simulink model "counter_test_16_ip"  (Simulink 6.2)
settings: Solver=ode45  StartTime=0.0  StopTime=6000  RelTol=1e-3
undefined symbols (not defined in the file or in its folder): iBOB
libraries: xbsIndex_r3 x81, xps_library x42, casper_library x11
settings Model: LastModifiedBy=tfiliba
settings DebuggingCC: SolverPrmCheckMsg=warning

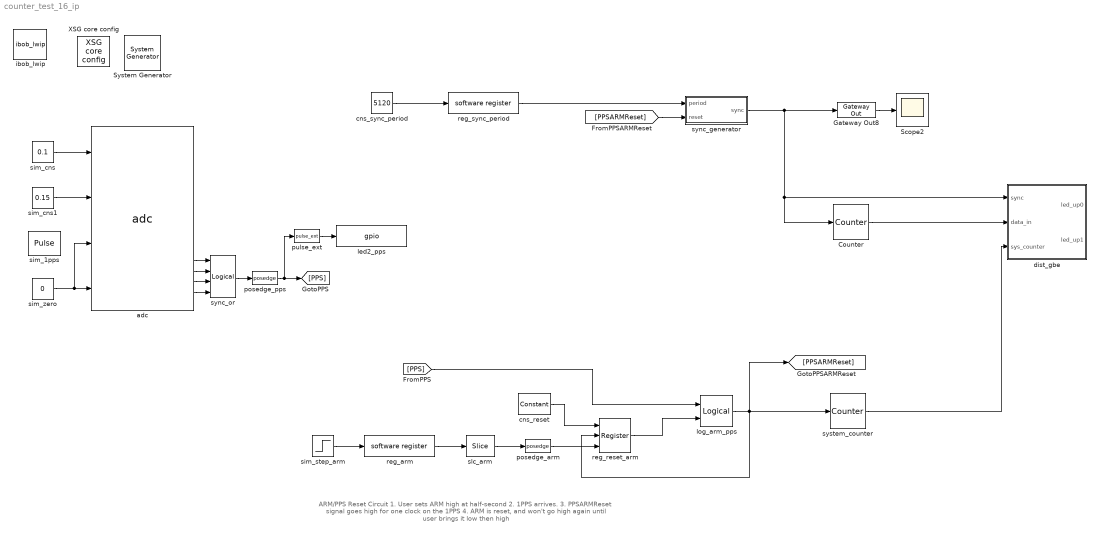
== system counter_test_16_ip ==
  note: ARM/PPS Reset Circuit
      | 1. User sets ARM high at half-second
      | 2. 1PPS arrives.
      | 3. PPSARMReset signal goes high for one clock on the 1PPS
      | 4. ARM is reset, and won't go high again until user brings it low then high
  " System Generator" : xbsIndex_r3/ System Generator  Tag=genX  xilinxfamily=Virtex2P  part=xc2vp50  speed=-7  package=ff1152  synthesis_tool=XST  directory=./counter_test_16_ip/sysgen  testbench=off  simulink_period=1  sysclk_period=5  incr_netlist=off  trim_vbits=Everywhere in SubSystem  dbl_ovrd=According to Block Masks  core_generation=According to Block Masks  run_coregen=off  deprecated_control=off  eval_field=0
      settings: AttributesFormatString=System\nGenerator
  Counter : xbsIndex_r3/Counter  cnt_type=Count Limited  n_bits=64  bin_pt=0  arith_type=Unsigned  start_count=0  cnt_to=15  cnt_by_val=1  operation=Up  explicit_period=on  period=1  load_pin=off  rst=on  en=off  dbl_ovrd=off  show_param=off  use_rpm=on  gen_core=off
      settings: xl_area=[0, 0, 0, 0, 0, 0, 0]
  Gateway Out8 : xbsIndex_r3/Gateway Out  output_type=Double  nbits=8  bin_pt=6  arith_type=Boolean  quantization=Truncate  overflow=Wrap  hdl_port=on  timing_constraint=None  locs_specified=off  LOCs={}  needs_fixed_name=off  show_param=off
      settings: xl_area=[0, 0, 0, 0, 0, 0, 0]
  Scope2 : Scope
      settings: YMin=-1  YMax=1  SaveName=ScopeData3
  XSG core config : xps_library/XSG core config  Tag=xps:xsg  hw_sys=iBOB  ibob_linux=off  clk_src=adc0_clk  gpio_clk_io_group=iBOB:sma  gpio_clk_bit_index=0  clk_rate=200  sample_period=1  synthesis_tool=XST  mpc_type=powerpc405
  adc : xps_library/adc  Tag=xps:adc  adc_brd=iBOB:adc0  adc_clk_rate=800  adc_interleave=off  sample_period=1
  cns_reset : xbsIndex_r3/Constant  const=1  equ=P=C  arith_type=Boolean  n_bits=1  bin_pt=0  opselect=C  inp2=PCIN>>17  opr=+  inp1=P  carry=CIN  iostate=0  explicit_period=on  period=1  dbl_ovrd=off
  cns_sync_period : Constant  Value=5120
  dist_gbe : Subsystem  mask(dist_gbe){numcomputers=16, numsamples=16, samplesperpacket=64}
      mask prompts: numcomputers "Num IPs (Must be power of 2)"; numsamples "Samples per spectrum (Number of clock cycles to generate 1 spectrum)"; samplesperpacket "Samples per packet (Number of samples to put in a packet)"
      mask init:
      | dist_gbe_init(gcb,...
      |     'numcomputers', numcomputers,...
      |     'numsamples', numsamples,...
      |     'samplesperpacket', samplesperpacket)
      settings: AttributesFormatString=IPs=16
  ibob_lwip : xps_library/ibob_lwip
  led2_pps : xps_library/gpio  Tag=xps:gpio  io_group=iBOB:led  io_dir=out  arith_type=Boolean  bitwidth=1  bin_pt=0  bit_index=3  sample_period=1  use_single_ended=off  use_ddr=off  reg_iob=on  reg_clk_phase=0  termination=None
  log_arm_pps : xbsIndex_r3/Logical  logical_function=AND  inputs=2  precision=Full  arith_type=Unsigned  n_bits=8  bin_pt=2  align_bp=on  latency=0  explicit_period=off  period=1  en=off  dbl_ovrd=off  show_param=off
      settings: xl_area=[0, 0, 0, 0, 0, 0, 0]
  posedge_arm : casper_library/Misc/posedge  Tag=Rising Edge Detector
  posedge_pps : casper_library/Misc/posedge  Tag=Rising Edge Detector
  pulse_ext : casper_library/Misc/pulse_ext  pulse_len=10000000
  reg_arm : xps_library/software register  Tag=xps:sw_reg  io_dir=From Processor  arith_type=Unsigned  bitwidth=32  bin_pt=0  sample_period=1  gw_name=counter_test_16_ip_reg_arm_user_data_out
  reg_reset_arm : xbsIndex_r3/Register  init=0  reg_only_valid=off  explicit_period=on  period=1  rst=on  en=on  out_en=off  dbl_ovrd=off  show_param=off
      settings: xl_area=[0, 0, 0, 0, 0, 0, 0]
  reg_sync_period : xps_library/software register  Tag=xps:sw_reg  io_dir=From Processor  arith_type=Unsigned  bitwidth=32  bin_pt=0  sample_period=1  gw_name=counter_test_16_ip_reg_sync_period_user_data_out
  sim_1pps : DiscretePulseGenerator  Period=1000  PulseWidth=3
  sim_cns : Constant  Value=0.1
  sim_cns1 : Constant  Value=0.15
  sim_step_arm : Step  SampleTime=0
  sim_zero : Constant  Value=0
  slc_arm : xbsIndex_r3/Slice  mode=Lower Bit Location + Width  nbits=1  bit1=0  base1=MSB of Input  bit0=0  base0=LSB of Input  boolean_output=on  explicit_period=off  period=1  dbl_ovrd=off
  sync_generator : Subsystem
  sync_or : xbsIndex_r3/Logical  logical_function=OR  inputs=4  precision=Full  arith_type=Unsigned  n_bits=8  bin_pt=2  align_bp=on  latency=1  explicit_period=off  period=1  en=off  dbl_ovrd=off  show_param=off
      settings: xl_area=[0, 0, 0, 0, 0, 0, 0]
  system_counter : xbsIndex_r3/Counter  cnt_type=Free Running  n_bits=64  bin_pt=0  arith_type=Unsigned  start_count=0  cnt_to=Inf  cnt_by_val=1  operation=Up  explicit_period=off  period=1  load_pin=off  rst=on  en=off  dbl_ovrd=off  show_param=off  use_rpm=on  gen_core=off
      settings: xl_area=[0, 0, 0, 0, 0, 0, 0]
  wires:
  reg_arm/1 -> slc_arm/1
  cns_reset/1 -> reg_reset_arm/1
  reg_reset_arm/1 -> log_arm_pps/2
  [PPS] -> log_arm_pps/1
  log_arm_pps/1 -> reg_reset_arm/2, system_counter/1, [PPSARMReset]
  slc_arm/1 -> posedge_arm/1
  posedge_arm/1 -> reg_reset_arm/3
  sim_step_arm/1 -> reg_arm/1
  reg_sync_period/1 -> sync_generator/1(period)
  sync_generator/1(sync) -> Gateway Out8/1, Counter/1, dist_gbe/1(sync)
  cns_sync_period/1 -> reg_sync_period/1
  Gateway Out8/1 -> Scope2/1
  [PPSARMReset] -> sync_generator/2(reset)
  sim_zero/1 -> adc/4, adc/3
  adc/13 -> sync_or/1
  adc/14 -> sync_or/2
  adc/15 -> sync_or/3
  adc/16 -> sync_or/4
  sync_or/1 -> posedge_pps/1
  posedge_pps/1 -> [PPS], pulse_ext/1
  pulse_ext/1 -> led2_pps/1
  sim_cns/1 -> adc/1
  sim_cns1/1 -> adc/2
  Counter/1 -> dist_gbe/2(data_in)
  system_counter/1 -> dist_gbe/3(sys_counter)

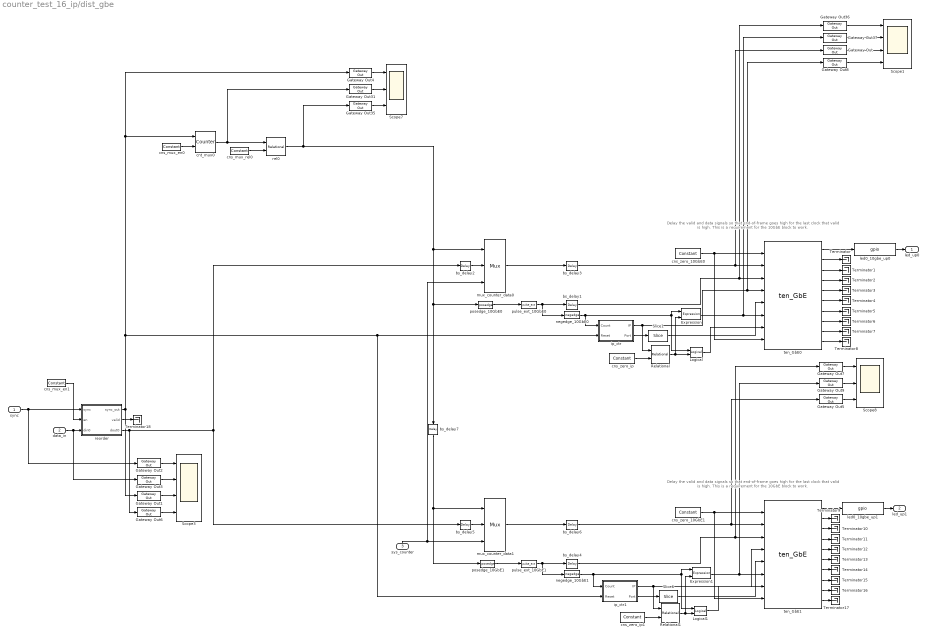
== system counter_test_16_ip/dist_gbe ==
  note: Delay the valid and data signals so that
      | end-of-frame goes high for the last clock
      | that valid is high. This is a requirement for
      | the 10GbE block to work.
  note: Delay the valid and data signals so that
      | end-of-frame goes high for the last clock
      | that valid is high. This is a requirement for
      | the 10GbE block to work.
  sync : Inport  Port=1  LatchInput=off
  data_in : Inport  Port=2  LatchInput=off
  sys_counter : Inport  Orientation=up  Port=3  LatchInput=off
  Expression : xbsIndex_r3/Expression  expression=a & ~b  precision=Full  arith_type=Unsigned  n_bits=8  bin_pt=2  align_bp=on  latency=0  explicit_period=off  period=1  en=off  dbl_ovrd=off  show_param=off
      settings: xl_area=[0, 0, 0, 0, 0, 0, 0]
  Expression1 : xbsIndex_r3/Expression  expression=a & ~b  precision=Full  arith_type=Unsigned  n_bits=8  bin_pt=2  align_bp=on  latency=0  explicit_period=off  period=1  en=off  dbl_ovrd=off  show_param=off
      settings: xl_area=[0, 0, 0, 0, 0, 0, 0]
  Gateway Out{,1..9,31,35..37} (14 alike) : xbsIndex_r3/Gateway Out  output_type=Double  nbits=8  bin_pt=6  arith_type=Boolean  quantization=Truncate  overflow=Wrap  hdl_port=on  timing_constraint=None  locs_specified=off  LOCs={}  needs_fixed_name=off  show_param=off
      settings: xl_area=[0, 0, 0, 0, 0, 0, 0]
  Logical : xbsIndex_r3/Logical  logical_function=AND  inputs=2  precision=Full  arith_type=Unsigned  n_bits=8  bin_pt=2  align_bp=on  latency=0  explicit_period=off  period=1  en=off  dbl_ovrd=off  show_param=off
      settings: xl_area=[0, 0, 0, 0, 0, 0, 0]
  Logical1 : xbsIndex_r3/Logical  logical_function=AND  inputs=2  precision=Full  arith_type=Unsigned  n_bits=8  bin_pt=2  align_bp=on  latency=0  explicit_period=off  period=1  en=off  dbl_ovrd=off  show_param=off
      settings: xl_area=[0, 0, 0, 0, 0, 0, 0]
  Relational : xbsIndex_r3/Relational  mode=a=b  latency=0  explicit_period=off  period=1  en=off  dbl_ovrd=off  show_param=off
      settings: xl_area=[0, 0, 0, 0, 0, 0, 0]
  Relational1 : xbsIndex_r3/Relational  mode=a=b  latency=0  explicit_period=off  period=1  en=off  dbl_ovrd=off  show_param=off
      settings: xl_area=[0, 0, 0, 0, 0, 0, 0]
  Scope1 : Scope  NumInputPorts=4
      settings: TimeRange=10000  YMin=0~0~-5~-5  YMax=1~1~40~5
  Scope3 : Scope  NumInputPorts=4
      settings: TimeRange=6000  YMin=0~0~-1~0  YMax=1~65~1~65  SaveName=ScopeData4
  Scope7 : Scope  NumInputPorts=3
      settings: YMin=0~0~0  YMax=1~275~1
  Scope8 : Scope  NumInputPorts=3
      settings: TimeRange=6000  YMin=0~0~0  YMax=1~1~5250  SaveName=ScopeData2
  Slice1 : xbsIndex_r3/Slice  mode=Lower Bit Location + Width  nbits=16  bit1=0  base1=MSB of Input  bit0=0  base0=LSB of Input  boolean_output=off  explicit_period=off  period=1  dbl_ovrd=off
  Slice6 : xbsIndex_r3/Slice  mode=Lower Bit Location + Width  nbits=16  bit1=0  base1=MSB of Input  bit0=0  base0=LSB of Input  boolean_output=off  explicit_period=off  period=1  dbl_ovrd=off
  Terminator{,1..18} (19 alike) : Terminator
  bs_delay{1..6} (6 alike) : xbsIndex_r3/Delay  latency=1  reg_retiming=off  explicit_period=on  period=1  en=off  accept_only_valid=off  init_zero=on  dbl_ovrd=off  show_param=off
      settings: xl_area=[0, 0, 0, 0, 0, 0, 0]
  bs_delay7 : xbsIndex_r3/Delay  Orientation=down  latency=64  reg_retiming=off  explicit_period=on  period=1  en=off  accept_only_valid=off  init_zero=on  dbl_ovrd=off  show_param=off
      settings: xl_area=[0, 0, 0, 0, 0, 0, 0]
  cns_mux_en0 : xbsIndex_r3/Constant  const=1  equ=P=C  arith_type=Boolean  n_bits=1  bin_pt=0  opselect=C  inp2=PCIN>>17  opr=+  inp1=P  carry=CIN  iostate=0  explicit_period=on  period=1  dbl_ovrd=off
  cns_mux_en1 : xbsIndex_r3/Constant  const=1  equ=P=C  arith_type=Boolean  n_bits=1  bin_pt=0  opselect=C  inp2=PCIN>>17  opr=+  inp1=P  carry=CIN  iostate=0  explicit_period=on  period=1  dbl_ovrd=off
  cns_mux_rel0 : xbsIndex_r3/Constant  const=127  equ=P=C  arith_type=Unsigned  n_bits=7  bin_pt=0  opselect=C  inp2=PCIN>>17  opr=+  inp1=P  carry=CIN  iostate=0  explicit_period=on  period=1  dbl_ovrd=off
  cns_zero_10GbE0 : xbsIndex_r3/Constant  const=0  equ=P=C  arith_type=Boolean  n_bits=32  bin_pt=0  opselect=C  inp2=PCIN>>17  opr=+  inp1=P  carry=CIN  iostate=0  explicit_period=on  period=1  dbl_ovrd=off
  cns_zero_10GbE1 : xbsIndex_r3/Constant  const=0  equ=P=C  arith_type=Boolean  n_bits=32  bin_pt=0  opselect=C  inp2=PCIN>>17  opr=+  inp1=P  carry=CIN  iostate=0  explicit_period=on  period=1  dbl_ovrd=off
  cns_zero_ip : xbsIndex_r3/Constant  const=0  equ=P=C  arith_type=Unsigned  n_bits=32  bin_pt=0  opselect=C  inp2=PCIN>>17  opr=+  inp1=P  carry=CIN  iostate=0  explicit_period=on  period=1  dbl_ovrd=off
  cns_zero_ip1 : xbsIndex_r3/Constant  const=0  equ=P=C  arith_type=Unsigned  n_bits=32  bin_pt=0  opselect=C  inp2=PCIN>>17  opr=+  inp1=P  carry=CIN  iostate=0  explicit_period=on  period=1  dbl_ovrd=off
  cnt_mux0 : xbsIndex_r3/Counter  cnt_type=Free Running  n_bits=7  bin_pt=0  arith_type=Unsigned  start_count=0  cnt_to=Inf  cnt_by_val=1  operation=Up  explicit_period=off  period=1  load_pin=off  rst=on  en=on  dbl_ovrd=off  show_param=off  use_rpm=on  gen_core=off
      settings: xl_area=[0, 0, 0, 0, 0, 0, 0]
  ip_ctr : Subsystem  mask(ip_ctr){numcomputers=8, odd_channels=1}
      mask prompts: numcomputers "Num IPs (Must be power of 2)"; odd_channels "Odd Channels"
      mask init:
      | ip_ctr_init(gcb,...
      |     'numcomputers',numcomputers,...
      |     'odd_channels',odd_channels)
      settings: AttributesFormatString=IPs=8
  ip_ctr1 : Subsystem  mask(ip_ctr){numcomputers=8, odd_channels=0}
      mask prompts: numcomputers "Num IPs (Must be power of 2)"; odd_channels "Odd Channels"
      mask init:
      | ip_ctr_init(gcb,...
      |     'numcomputers',numcomputers,...
      |     'odd_channels',odd_channels)
      settings: AttributesFormatString=IPs=8
  led0_10gbe_up0 : xps_library/gpio  Tag=xps:gpio  io_group=iBOB:led  io_dir=out  arith_type=Boolean  bitwidth=1  bin_pt=0  bit_index=1  sample_period=1  use_single_ended=off  use_ddr=off  reg_iob=on  reg_clk_phase=0  termination=None
  led0_10gbe_up1 : xps_library/gpio  Tag=xps:gpio  io_group=iBOB:led  io_dir=out  arith_type=Boolean  bitwidth=1  bin_pt=0  bit_index=2  sample_period=1  use_single_ended=off  use_ddr=off  reg_iob=on  reg_clk_phase=0  termination=None
  mux_counter_data0 : xbsIndex_r3/Mux  inputs=2  precision=Full  arith_type="Signed  (2's comp)"  n_bits=8  bin_pt=2  quantization=Truncate  overflow=Wrap  latency=1  explicit_period=off  period=1  en=off  dbl_ovrd=off  show_param=off  mux_type=off  use_rpm=off  gen_core=off
      settings: xl_area=[0, 0, 0, 0, 0, 0, 0]
  mux_counter_data1 : xbsIndex_r3/Mux  inputs=2  precision=Full  arith_type="Signed  (2's comp)"  n_bits=8  bin_pt=2  quantization=Truncate  overflow=Wrap  latency=1  explicit_period=off  period=1  en=off  dbl_ovrd=off  show_param=off  mux_type=off  use_rpm=off  gen_core=off
      settings: xl_area=[0, 0, 0, 0, 0, 0, 0]
  negedge_10GbE0 : casper_library/Misc/negedge  Tag=Rising Edge Detector
  negedge_10GbE1 : casper_library/Misc/negedge  Tag=Rising Edge Detector
  posedge_10GbE0 : casper_library/Misc/posedge  Tag=Rising Edge Detector
  posedge_10GbE1 : casper_library/Misc/posedge  Tag=Rising Edge Detector
  pulse_ext_10GbE0 : casper_library/Misc/pulse_ext  pulse_len=65
  pulse_ext_10GbE1 : casper_library/Misc/pulse_ext  pulse_len=65
  rel0 : xbsIndex_r3/Relational  mode=a=b  latency=1  explicit_period=off  period=1  en=off  dbl_ovrd=off  show_param=off
      settings: xl_area=[0, 0, 0, 0, 0, 0, 0]
  reorder : Subsystem  AncestorBlock=casper_library/Reorder/reorder  mask(reorder){map=[0 16 32 48 64 80 96 112 128 144 160 176 192 208 224 240 256 272 288 304 320 336 352 368 384 400 416 432 448 464 480 496 512 528 544 560 576 592 608 624 640 656 672 688 704 720 736 752 768 784 800 816 832 848 864 880 896 912 928 944 960 976 992 1008 1 17 33 49 65 81 97 113 129 145 161 177 193 209 225 241 257 273 289 305 321 337 353 369 385 401 417 433 449 465 481 497 513 529 545 561 577 593 609 625 641 657 673 689 705 721 737 753 769 785 801 817 833 849 865 881 897 913 929 945 961 977 993 1009 2 18 34 50 66 82 98 114 130 146 162 178 194 210 226 242 258 274 290 306 322 338 354 370 386 402 418 434 450 466 482 498 514 530 546 562 578 594 610 626 642 658 674 690 706 722 738 754 770 786 802 818 834 850 866 882 898 914 930 946 962 978 994 1010 3 19 35 51 67 83 99 115 131 147 163 179 195 211 227 243 259 275 291 307 323 339 355 371 387 403 419 435 451 467 483 499 515 531 547 563 579 595 611 627 643 659 675 691 707 723 739 755 771 787 803 819 835 851 867 883 899 915 931 947 963 979 995 1011 4 20 36 52 68 84 100 116 132 148 164 180 196 212 228 244 260 276 292 308 324 340 356 372 388 404 420 436 452 468 484 500 516 532 548 564 580 596 612 628 644 660 676 692 708 724 740 756 772 788 804 820 836 852 868 884 900 916 932 948 964 980 996 1012 5 21 37 53 69 85 101 117 133 149 165 181 197 213 229 245 261 277 293 309 325 341 357 373 389 405 421 437 453 469 485 501 517 533 549 565 581 597 613 629 645 661 677 693 709 725 741 757 773 789 805 821 837 853 869 885 901 917 933 949 965 981 997 1013 6 22 38 54 70 86 102 118 134 150 166 182 198 214 230 246 262 278 294 310 326 342 358 374 390 406 422 438 454 470 486 502 518 534 550 566 582 598 614 630 646 662 678 694 710 726 742 758 774 790 806 822 838 854 870 886 902 918 934 950 966 982 998 1014 7 23 39 55 71 87 103 119 135 151 167 183 199 215 231 247 263 279 295 311 327 343 359 375 391 407 423 439 455 471 487 503 519 535 551 567 583 599 615 631 647 663 679 695 711 727 743 759 775 791 807 823 839 855 871 887 903 919 935 951 967 983 999 1015 8 24 40 56 72 88 104 120 136 152 168 184 200 216 232 248 264 280 296 312 328 344 360 376 392 408 424 440 456 472 488 504 520 536 552 568 584 600 616 632 648 664 680 696 712 728 744 760 776 792 808 824 840 856 872 888 904 920 936 952 968 984 1000 1016 9 25 41 57 73 89 105 121 137 153 169 185 201 217 233 249 265 281 297 313 329 345 361 377 393 409 425 441 457 473 489 505 521 537 553 569 585 601 617 633 649 665 681 697 713 729 745 761 777 793 809 825 841 857 873 889 905 921 937 953 969 985 1001 1017 10 26 42 58 74 90 106 122 138 154 170 186 202 218 234 250 266 282 298 314 330 346 362 378 394 410 426 442 458 474 490 506 522 538 554 570 586 602 618 634 650 666 682 698 714 730 746 762 778 794 810 826 842 858 874 890 906 922 938 954 970 986 1002 1018 11 27 43 59 75 91 107 123 139 155 171 187 203 219 235 251 267 283 299 315 331 347 363 379 395 411 427 443 459 475 491 507 523 539 555 571 587 603 619 635 651 667 683 699 715 731 747 763 779 795 811 827 843 859 875 891 907 923 939 955 971 987 1003 1019 12 28 44 60 76 92 108 124 140 156 172 188 204 220 236 252 268 284 300 316 332 348 364 380 396 412 428 444 460 476 492 508 524 540 556 572 588 604 620 636 652 668 684 700 716 732 748 764 780 796 812 828 844 860 876 892 908 924 940 956 972 988 1004 1020 13 29 45 61 77 93 109 125 141 157 173 189 205 221 237 253 269 285 301 317 333 349 365 381 397 413 429 445 461 477 493 509 525 541 557 573 589 605 621 637 653 669 685 701 717 733 749 765 781 797 813 829 845 861 877 893 909 925 941 957 973 989 1005 1021 14 30 46 62 78 94 110 126 142 158 174 190 206 222 238 254 270 286 302 318 334 350 366 382 398 414 430 446 462 478 494 510 526 542 558 574 590 606 622 638 654 670 686 702 718 734 750 766 782 798 814 830 846 862 878 894 910 926 942 958 974 990 1006 1022 15 31 47 63 79 95 111 127 143 159 175 191 207 223 239 255 271 287 303 319 335 351 367 383 399 415 431 447 463 479 495 511 527 543 559 575 591 607 623 639 655 671 687 703 719 735 751 767 783 799 815 831 847 863 879 895 911 927 943 959 975 991 1007 1023], n_inputs=1, bram_latency=2, map_latency=1, double_buffer=0}
      mask prompts: map "Output Order:"; n_inputs "Number of inputs"; bram_latency "BRAM Latency"; map_latency "Map Latency"; double_buffer "Double Buffer"
      mask init:
      | reorder_init(gcb, ...
      |     'map', map, ...
      |     'n_inputs', n_inputs, ...
      |     'bram_latency', bram_latency, ...
      |     'map_latency', map_latency, ...
      |     'double_buffer', double_buffer);
      settings: AttributesFormatString=order=5
  ten_GbE0 : xps_library/ten_GbE  Tag=xps:tengbe  port=iBOB:0  mac_lite=on  show_param=on  pre_emph=2  swing=800
  ten_GbE1 : xps_library/ten_GbE  Tag=xps:tengbe  port=iBOB:1  mac_lite=on  show_param=on  pre_emph=2  swing=800
  led_up0 : Outport
  led_up1 : Outport  Port=2
  wires:
  sys_counter/1 -> mux_counter_data1/3, mux_counter_data0/3
  data_in/1 -> Gateway Out3/1, reorder/3(din0)
  reorder/2(valid) -> Terminator18/1
  Gateway Out36/1 -> Scope1/1
  ten_GbE1/10 -> Terminator17/1
  ten_GbE1/9 -> Terminator16/1
  ten_GbE1/8 -> Terminator15/1
  ten_GbE1/7 -> Terminator14/1
  ten_GbE1/6 -> Terminator13/1
  ten_GbE1/5 -> Terminator12/1
  ten_GbE1/4 -> Terminator11/1
  ten_GbE1/3 -> Terminator10/1
  ten_GbE1/2 -> Terminator9/1
  ten_GbE0/10 -> Terminator8/1
  ten_GbE0/9 -> Terminator7/1
  ten_GbE0/8 -> Terminator6/1
  ten_GbE0/7 -> Terminator5/1
  ten_GbE0/6 -> Terminator4/1
  ten_GbE0/5 -> Terminator3/1
  ten_GbE0/4 -> Terminator2/1
  ten_GbE0/3 -> Terminator1/1
  ten_GbE0/2 -> Terminator/1
  ten_GbE0/1 -> led0_10gbe_up0/1
  cns_zero_10GbE0/1 -> ten_GbE0/1, ten_GbE0/8
  mux_counter_data0/1 -> bs_delay3/1
  cnt_mux0/1 -> rel0/1, Gateway Out31/1
  cns_mux_en0/1 -> cnt_mux0/2
  Gateway Out37/1 -> Scope1/2
  Gateway Out/1 -> Scope1/3
  pulse_ext_10GbE0/1 -> bs_delay1/1, negedge_10GbE0/1
  negedge_10GbE0/1 -> Logical/1, Expression/1, ip_ctr/1(Count)
  cns_mux_rel0/1 -> rel0/2
  rel0/1 -> mux_counter_data0/1, posedge_10GbE0/1, bs_delay7/1, Gateway Out35/1
  posedge_10GbE0/1 -> pulse_ext_10GbE0/1
  bs_delay1/1 -> ten_GbE0/3, Gateway Out36/1
  bs_delay3/1 -> ten_GbE0/2, Gateway Out/1
  Gateway Out4/1 -> Scope7/1
  Gateway Out31/1 -> Scope7/2
  Gateway Out35/1 -> Scope7/3
  bs_delay2/1 -> mux_counter_data0/2
  ten_GbE1/1 -> led0_10gbe_up1/1
  cns_zero_10GbE1/1 -> ten_GbE1/1, ten_GbE1/8
  mux_counter_data1/1 -> bs_delay6/1
  pulse_ext_10GbE1/1 -> negedge_10GbE1/1, bs_delay4/1
  negedge_10GbE1/1 -> Logical1/1, Expression1/1, ip_ctr1/1(Count)
  posedge_10GbE1/1 -> pulse_ext_10GbE1/1
  bs_delay4/1 -> ten_GbE1/3, Gateway Out7/1
  bs_delay6/1 -> ten_GbE1/2, Gateway Out5/1
  bs_delay5/1 -> mux_counter_data1/2
  bs_delay7/1 -> mux_counter_data1/1, posedge_10GbE1/1
  Gateway Out7/1 -> Scope8/1
  Gateway Out9/1 -> Scope8/2
  Gateway Out5/1 -> Scope8/3
  reorder/3(dout0) -> bs_delay5/1, bs_delay2/1, Gateway Out6/1
  cns_mux_en1/1 -> reorder/2(en)
  Gateway Out2/1 -> Scope3/1
  Gateway Out3/1 -> Scope3/2
  Gateway Out1/1 -> Scope3/3
  Gateway Out6/1 -> Scope3/4
  reorder/1(sync_out) -> Gateway Out1/1, cnt_mux0/1, Gateway Out4/1, ip_ctr/2(Reset), ip_ctr1/2(Reset)
  ip_ctr/1(IP) -> Relational/1, ten_GbE0/4, Gateway Out8/1
  sync/1 -> reorder/1(sync), Gateway Out2/1
  led0_10gbe_up0/1 -> led_up0/1
  led0_10gbe_up1/1 -> led_up1/1
  cns_zero_ip/1 -> Relational/2
  Logical/1 -> ten_GbE0/7
  Relational/1 -> Logical/2, Expression/2
  Expression/1 -> ten_GbE0/6, Gateway Out37/1
  ip_ctr1/1(IP) -> Relational1/1, ten_GbE1/4
  Relational1/1 -> Logical1/2, Expression1/2
  Logical1/1 -> ten_GbE1/7
  Expression1/1 -> ten_GbE1/6, Gateway Out9/1
  cns_zero_ip1/1 -> Relational1/2
  Gateway Out8/1 -> Scope1/4
  ip_ctr/2(Port) -> Slice1/1
  Slice1/1 -> ten_GbE0/5
  ip_ctr1/2(Port) -> Slice6/1
  Slice6/1 -> ten_GbE1/5

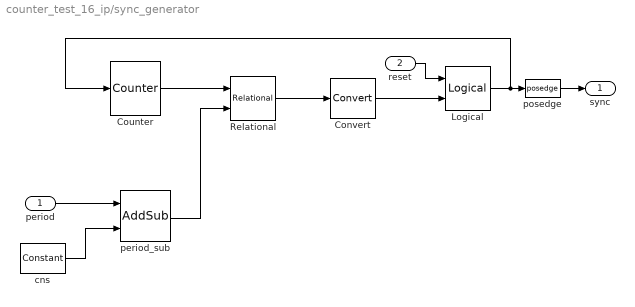
== system counter_test_16_ip/sync_generator ==
  period : Inport  Port=1  LatchInput=off
  reset : Inport  Port=2  LatchInput=off
  Convert : xbsIndex_r3/Convert  arith_type=Boolean  n_bits=8  bin_pt=6  quantization=Truncate  overflow=Wrap  latency=1  explicit_period=off  period=1  dbl_ovrd=off  show_param=off  inserted_by_tool=off  pipeline=off
      settings: xl_area=[0, 0, 0, 0, 0, 0, 0]
  Counter : xbsIndex_r3/Counter  cnt_type=Free Running  n_bits=32  bin_pt=0  arith_type=Unsigned  start_count=1  cnt_to=Inf  cnt_by_val=1  operation=Up  explicit_period=on  period=1  load_pin=off  rst=on  en=off  dbl_ovrd=off  show_param=off  use_rpm=on  gen_core=off
      settings: xl_area=[0, 0, 0, 0, 0, 0, 0]
  Logical : xbsIndex_r3/Logical  logical_function=OR  inputs=2  precision=Full  arith_type=Unsigned  n_bits=8  bin_pt=2  align_bp=on  latency=0  explicit_period=off  period=1  en=off  dbl_ovrd=off  show_param=off
      settings: xl_area=[0, 0, 0, 0, 0, 0, 0]
  Relational : xbsIndex_r3/Relational  mode=a>=b  latency=1  explicit_period=off  period=1  en=off  dbl_ovrd=off  show_param=off
      settings: xl_area=[0, 0, 0, 0, 0, 0, 0]
  cns : xbsIndex_r3/Constant  const=4  equ=P=C  arith_type=Unsigned  n_bits=3  bin_pt=0  opselect=C  inp2=PCIN>>17  opr=+  inp1=P  carry=CIN  iostate=0  explicit_period=on  period=1  dbl_ovrd=off
  period_sub : xbsIndex_r3/AddSub  mode=Subtraction  precision=User Defined  arith_type=Unsigned  n_bits=32  bin_pt=0  quantization=Truncate  overflow=Wrap  latency=0  explicit_period=off  period=1  use_carryin=off  use_carryout=off  en=off  dbl_ovrd=off  show_param=off  use_core=on  pipeline=off  use_rpm=on  gen_core=off
      settings: xl_area=[0, 0, 0, 0, 0, 0, 0]
  posedge : casper_library/Misc/posedge  Tag=Rising Edge Detector
  sync : Outport
  wires:
  Counter/1 -> Relational/1
  Relational/1 -> Convert/1
  Convert/1 -> Logical/2
  Logical/1 -> Counter/1, posedge/1
  reset/1 -> Logical/1
  period/1 -> period_sub/1
  period_sub/1 -> Relational/2
  cns/1 -> period_sub/2
  posedge/1 -> sync/1

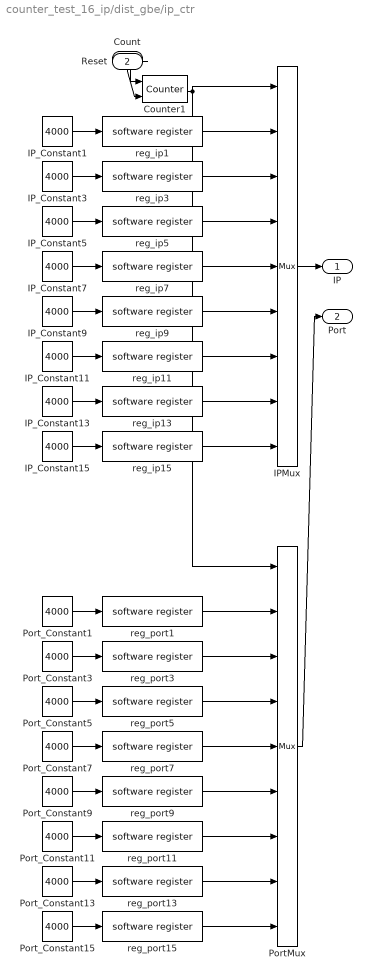
== system counter_test_16_ip/dist_gbe/ip_ctr ==
  Count : Inport  Orientation=down  Port=1  LatchInput=off
  Reset : Inport  Port=2  LatchInput=off
  Counter1 : xbsIndex_r3/Counter  cnt_type=Free Running  n_bits=3  bin_pt=0  arith_type=Unsigned  start_count=0  cnt_to=Inf  cnt_by_val=1  operation=Up  explicit_period=off  period=1  load_pin=off  rst=on  en=on  dbl_ovrd=off  show_param=off  use_rpm=on  gen_core=off
      settings: xl_area=[0, 0, 0, 0, 0, 0, 0]
  IPMux : xbsIndex_r3/Mux  inputs=8  precision=Full  arith_type="Signed  (2's comp)"  n_bits=8  bin_pt=2  quantization=Truncate  overflow=Wrap  latency=0  explicit_period=off  period=1  en=off  dbl_ovrd=off  show_param=off  mux_type=off  use_rpm=off  gen_core=off
      settings: xl_area=[0, 0, 0, 0, 0, 0, 0]
  IP_Constant{1,3,5,7,9,11,13,15} (8 alike) : Constant  Value=4000
  PortMux : xbsIndex_r3/Mux  inputs=8  precision=Full  arith_type="Signed  (2's comp)"  n_bits=8  bin_pt=2  quantization=Truncate  overflow=Wrap  latency=0  explicit_period=off  period=1  en=off  dbl_ovrd=off  show_param=off  mux_type=off  use_rpm=off  gen_core=off
      settings: xl_area=[0, 0, 0, 0, 0, 0, 0]
  Port_Constant{1,3,5,7,9,11,13,15} (8 alike) : Constant  Value=4000
  reg_ip1 : xps_library/software register  Tag=xps:sw_reg  io_dir=From Processor  arith_type=Unsigned  bitwidth=32  bin_pt=0  sample_period=1  gw_name=counter_test_16_ip_dist_gbe_ip_ctr_reg_ip1_user_data_out
  reg_ip11 : xps_library/software register  Tag=xps:sw_reg  io_dir=From Processor  arith_type=Unsigned  bitwidth=32  bin_pt=0  sample_period=1  gw_name=counter_test_16_ip_dist_gbe_ip_ctr_reg_ip11_user_data_out
  reg_ip13 : xps_library/software register  Tag=xps:sw_reg  io_dir=From Processor  arith_type=Unsigned  bitwidth=32  bin_pt=0  sample_period=1  gw_name=counter_test_16_ip_dist_gbe_ip_ctr_reg_ip13_user_data_out
  reg_ip15 : xps_library/software register  Tag=xps:sw_reg  io_dir=From Processor  arith_type=Unsigned  bitwidth=32  bin_pt=0  sample_period=1  gw_name=counter_test_16_ip_dist_gbe_ip_ctr_reg_ip15_user_data_out
  reg_ip3 : xps_library/software register  Tag=xps:sw_reg  io_dir=From Processor  arith_type=Unsigned  bitwidth=32  bin_pt=0  sample_period=1  gw_name=counter_test_16_ip_dist_gbe_ip_ctr_reg_ip3_user_data_out
  reg_ip5 : xps_library/software register  Tag=xps:sw_reg  io_dir=From Processor  arith_type=Unsigned  bitwidth=32  bin_pt=0  sample_period=1  gw_name=counter_test_16_ip_dist_gbe_ip_ctr_reg_ip5_user_data_out
  reg_ip7 : xps_library/software register  Tag=xps:sw_reg  io_dir=From Processor  arith_type=Unsigned  bitwidth=32  bin_pt=0  sample_period=1  gw_name=counter_test_16_ip_dist_gbe_ip_ctr_reg_ip7_user_data_out
  reg_ip9 : xps_library/software register  Tag=xps:sw_reg  io_dir=From Processor  arith_type=Unsigned  bitwidth=32  bin_pt=0  sample_period=1  gw_name=counter_test_16_ip_dist_gbe_ip_ctr_reg_ip9_user_data_out
  reg_port1 : xps_library/software register  Tag=xps:sw_reg  io_dir=From Processor  arith_type=Unsigned  bitwidth=32  bin_pt=0  sample_period=1  gw_name=counter_test_16_ip_dist_gbe_ip_ctr_reg_port1_user_data_out
  reg_port11 : xps_library/software register  Tag=xps:sw_reg  io_dir=From Processor  arith_type=Unsigned  bitwidth=32  bin_pt=0  sample_period=1  gw_name=counter_test_16_ip_dist_gbe_ip_ctr_reg_port11_user_data_out
  reg_port13 : xps_library/software register  Tag=xps:sw_reg  io_dir=From Processor  arith_type=Unsigned  bitwidth=32  bin_pt=0  sample_period=1  gw_name=counter_test_16_ip_dist_gbe_ip_ctr_reg_port13_user_data_out
  reg_port15 : xps_library/software register  Tag=xps:sw_reg  io_dir=From Processor  arith_type=Unsigned  bitwidth=32  bin_pt=0  sample_period=1  gw_name=counter_test_16_ip_dist_gbe_ip_ctr_reg_port15_user_data_out
  reg_port3 : xps_library/software register  Tag=xps:sw_reg  io_dir=From Processor  arith_type=Unsigned  bitwidth=32  bin_pt=0  sample_period=1  gw_name=counter_test_16_ip_dist_gbe_ip_ctr_reg_port3_user_data_out
  reg_port5 : xps_library/software register  Tag=xps:sw_reg  io_dir=From Processor  arith_type=Unsigned  bitwidth=32  bin_pt=0  sample_period=1  gw_name=counter_test_16_ip_dist_gbe_ip_ctr_reg_port5_user_data_out
  reg_port7 : xps_library/software register  Tag=xps:sw_reg  io_dir=From Processor  arith_type=Unsigned  bitwidth=32  bin_pt=0  sample_period=1  gw_name=counter_test_16_ip_dist_gbe_ip_ctr_reg_port7_user_data_out
  reg_port9 : xps_library/software register  Tag=xps:sw_reg  io_dir=From Processor  arith_type=Unsigned  bitwidth=32  bin_pt=0  sample_period=1  gw_name=counter_test_16_ip_dist_gbe_ip_ctr_reg_port9_user_data_out
  IP : Outport
  Port : Outport  Port=2
  wires:
  Reset/1 -> Counter1/1
  Count/1 -> Counter1/2
  Counter1/1 -> IPMux/1, PortMux/1
  IPMux/1 -> IP/1
  PortMux/1 -> Port/1
  IP_Constant1/1 -> reg_ip1/1
  reg_ip1/1 -> IPMux/2
  Port_Constant1/1 -> reg_port1/1
  reg_port1/1 -> PortMux/2
  IP_Constant3/1 -> reg_ip3/1
  reg_ip3/1 -> IPMux/3
  Port_Constant3/1 -> reg_port3/1
  reg_port3/1 -> PortMux/3
  IP_Constant5/1 -> reg_ip5/1
  reg_ip5/1 -> IPMux/4
  Port_Constant5/1 -> reg_port5/1
  reg_port5/1 -> PortMux/4
  IP_Constant7/1 -> reg_ip7/1
  reg_ip7/1 -> IPMux/5
  Port_Constant7/1 -> reg_port7/1
  reg_port7/1 -> PortMux/5
  IP_Constant9/1 -> reg_ip9/1
  reg_ip9/1 -> IPMux/6
  Port_Constant9/1 -> reg_port9/1
  reg_port9/1 -> PortMux/6
  IP_Constant11/1 -> reg_ip11/1
  reg_ip11/1 -> IPMux/7
  Port_Constant11/1 -> reg_port11/1
  reg_port11/1 -> PortMux/7
  IP_Constant13/1 -> reg_ip13/1
  reg_ip13/1 -> IPMux/8
  Port_Constant13/1 -> reg_port13/1
  reg_port13/1 -> PortMux/8
  IP_Constant15/1 -> reg_ip15/1
  reg_ip15/1 -> IPMux/9
  Port_Constant15/1 -> reg_port15/1
  reg_port15/1 -> PortMux/9

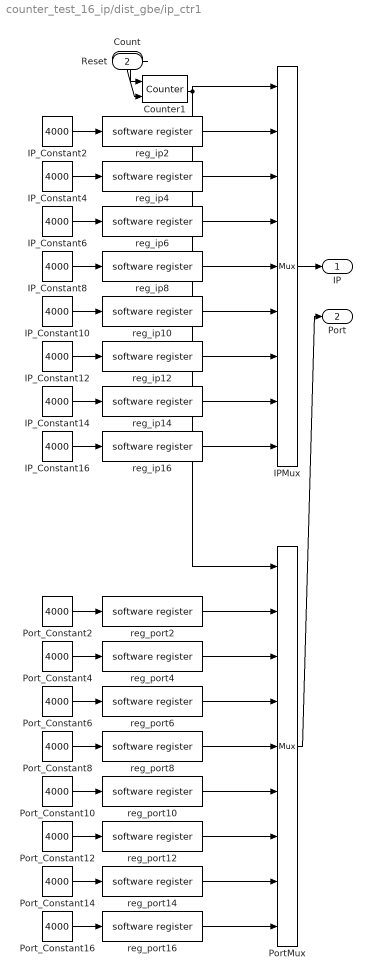
== system counter_test_16_ip/dist_gbe/ip_ctr1 ==
  Count : Inport  Orientation=down  Port=1  LatchInput=off
  Reset : Inport  Port=2  LatchInput=off
  Counter1 : xbsIndex_r3/Counter  cnt_type=Free Running  n_bits=3  bin_pt=0  arith_type=Unsigned  start_count=0  cnt_to=Inf  cnt_by_val=1  operation=Up  explicit_period=off  period=1  load_pin=off  rst=on  en=on  dbl_ovrd=off  show_param=off  use_rpm=on  gen_core=off
      settings: xl_area=[0, 0, 0, 0, 0, 0, 0]
  IPMux : xbsIndex_r3/Mux  inputs=8  precision=Full  arith_type="Signed  (2's comp)"  n_bits=8  bin_pt=2  quantization=Truncate  overflow=Wrap  latency=0  explicit_period=off  period=1  en=off  dbl_ovrd=off  show_param=off  mux_type=off  use_rpm=off  gen_core=off
      settings: xl_area=[0, 0, 0, 0, 0, 0, 0]
  IP_Constant{2,4,6,8,10,12,14,16} (8 alike) : Constant  Value=4000
  PortMux : xbsIndex_r3/Mux  inputs=8  precision=Full  arith_type="Signed  (2's comp)"  n_bits=8  bin_pt=2  quantization=Truncate  overflow=Wrap  latency=0  explicit_period=off  period=1  en=off  dbl_ovrd=off  show_param=off  mux_type=off  use_rpm=off  gen_core=off
      settings: xl_area=[0, 0, 0, 0, 0, 0, 0]
  Port_Constant{2,4,6,8,10,12,14,16} (8 alike) : Constant  Value=4000
  reg_ip10 : xps_library/software register  Tag=xps:sw_reg  io_dir=From Processor  arith_type=Unsigned  bitwidth=32  bin_pt=0  sample_period=1  gw_name=counter_test_16_ip_dist_gbe_ip_ctr1_reg_ip10_user_data_out
  reg_ip12 : xps_library/software register  Tag=xps:sw_reg  io_dir=From Processor  arith_type=Unsigned  bitwidth=32  bin_pt=0  sample_period=1  gw_name=counter_test_16_ip_dist_gbe_ip_ctr1_reg_ip12_user_data_out
  reg_ip14 : xps_library/software register  Tag=xps:sw_reg  io_dir=From Processor  arith_type=Unsigned  bitwidth=32  bin_pt=0  sample_period=1  gw_name=counter_test_16_ip_dist_gbe_ip_ctr1_reg_ip14_user_data_out
  reg_ip16 : xps_library/software register  Tag=xps:sw_reg  io_dir=From Processor  arith_type=Unsigned  bitwidth=32  bin_pt=0  sample_period=1  gw_name=counter_test_16_ip_dist_gbe_ip_ctr1_reg_ip16_user_data_out
  reg_ip2 : xps_library/software register  Tag=xps:sw_reg  io_dir=From Processor  arith_type=Unsigned  bitwidth=32  bin_pt=0  sample_period=1  gw_name=counter_test_16_ip_dist_gbe_ip_ctr1_reg_ip2_user_data_out
  reg_ip4 : xps_library/software register  Tag=xps:sw_reg  io_dir=From Processor  arith_type=Unsigned  bitwidth=32  bin_pt=0  sample_period=1  gw_name=counter_test_16_ip_dist_gbe_ip_ctr1_reg_ip4_user_data_out
  reg_ip6 : xps_library/software register  Tag=xps:sw_reg  io_dir=From Processor  arith_type=Unsigned  bitwidth=32  bin_pt=0  sample_period=1  gw_name=counter_test_16_ip_dist_gbe_ip_ctr1_reg_ip6_user_data_out
  reg_ip8 : xps_library/software register  Tag=xps:sw_reg  io_dir=From Processor  arith_type=Unsigned  bitwidth=32  bin_pt=0  sample_period=1  gw_name=counter_test_16_ip_dist_gbe_ip_ctr1_reg_ip8_user_data_out
  reg_port10 : xps_library/software register  Tag=xps:sw_reg  io_dir=From Processor  arith_type=Unsigned  bitwidth=32  bin_pt=0  sample_period=1  gw_name=counter_test_16_ip_dist_gbe_ip_ctr1_reg_port10_user_data_out
  reg_port12 : xps_library/software register  Tag=xps:sw_reg  io_dir=From Processor  arith_type=Unsigned  bitwidth=32  bin_pt=0  sample_period=1  gw_name=counter_test_16_ip_dist_gbe_ip_ctr1_reg_port12_user_data_out
  reg_port14 : xps_library/software register  Tag=xps:sw_reg  io_dir=From Processor  arith_type=Unsigned  bitwidth=32  bin_pt=0  sample_period=1  gw_name=counter_test_16_ip_dist_gbe_ip_ctr1_reg_port14_user_data_out
  reg_port16 : xps_library/software register  Tag=xps:sw_reg  io_dir=From Processor  arith_type=Unsigned  bitwidth=32  bin_pt=0  sample_period=1  gw_name=counter_test_16_ip_dist_gbe_ip_ctr1_reg_port16_user_data_out
  reg_port2 : xps_library/software register  Tag=xps:sw_reg  io_dir=From Processor  arith_type=Unsigned  bitwidth=32  bin_pt=0  sample_period=1  gw_name=counter_test_16_ip_dist_gbe_ip_ctr1_reg_port2_user_data_out
  reg_port4 : xps_library/software register  Tag=xps:sw_reg  io_dir=From Processor  arith_type=Unsigned  bitwidth=32  bin_pt=0  sample_period=1  gw_name=counter_test_16_ip_dist_gbe_ip_ctr1_reg_port4_user_data_out
  reg_port6 : xps_library/software register  Tag=xps:sw_reg  io_dir=From Processor  arith_type=Unsigned  bitwidth=32  bin_pt=0  sample_period=1  gw_name=counter_test_16_ip_dist_gbe_ip_ctr1_reg_port6_user_data_out
  reg_port8 : xps_library/software register  Tag=xps:sw_reg  io_dir=From Processor  arith_type=Unsigned  bitwidth=32  bin_pt=0  sample_period=1  gw_name=counter_test_16_ip_dist_gbe_ip_ctr1_reg_port8_user_data_out
  IP : Outport
  Port : Outport  Port=2
  wires:
  Reset/1 -> Counter1/1
  Count/1 -> Counter1/2
  Counter1/1 -> IPMux/1, PortMux/1
  IPMux/1 -> IP/1
  PortMux/1 -> Port/1
  IP_Constant2/1 -> reg_ip2/1
  reg_ip2/1 -> IPMux/2
  Port_Constant2/1 -> reg_port2/1
  reg_port2/1 -> PortMux/2
  IP_Constant4/1 -> reg_ip4/1
  reg_ip4/1 -> IPMux/3
  Port_Constant4/1 -> reg_port4/1
  reg_port4/1 -> PortMux/3
  IP_Constant6/1 -> reg_ip6/1
  reg_ip6/1 -> IPMux/4
  Port_Constant6/1 -> reg_port6/1
  reg_port6/1 -> PortMux/4
  IP_Constant8/1 -> reg_ip8/1
  reg_ip8/1 -> IPMux/5
  Port_Constant8/1 -> reg_port8/1
  reg_port8/1 -> PortMux/5
  IP_Constant10/1 -> reg_ip10/1
  reg_ip10/1 -> IPMux/6
  Port_Constant10/1 -> reg_port10/1
  reg_port10/1 -> PortMux/6
  IP_Constant12/1 -> reg_ip12/1
  reg_ip12/1 -> IPMux/7
  Port_Constant12/1 -> reg_port12/1
  reg_port12/1 -> PortMux/7
  IP_Constant14/1 -> reg_ip14/1
  reg_ip14/1 -> IPMux/8
  Port_Constant14/1 -> reg_port14/1
  reg_port14/1 -> PortMux/8
  IP_Constant16/1 -> reg_ip16/1
  reg_ip16/1 -> IPMux/9
  Port_Constant16/1 -> reg_port16/1
  reg_port16/1 -> PortMux/9

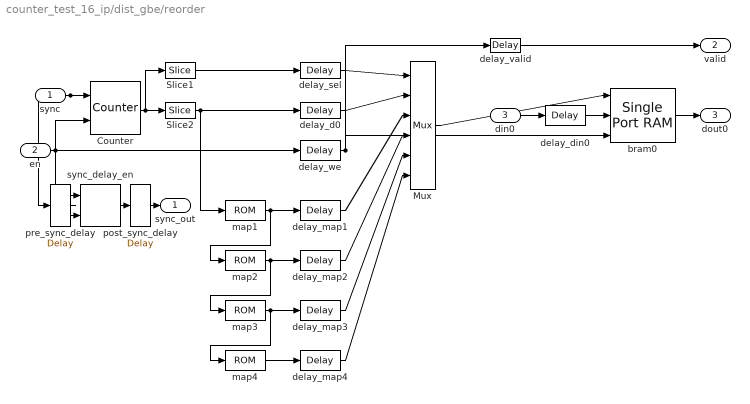
== system counter_test_16_ip/dist_gbe/reorder ==
  sync : Inport  Port=1  LatchInput=off
  en : Inport  Port=2  LatchInput=off
  din0 : Inport  Port=3  LatchInput=off
  Counter : xbsIndex_r3/Counter  cnt_type=Count Limited  n_bits=13  bin_pt=0  arith_type=Unsigned  start_count=0  cnt_to=5119  cnt_by_val=1  operation=Up  explicit_period=off  period=1  load_pin=off  rst=on  en=on  dbl_ovrd=off  show_param=off  use_rpm=on  gen_core=off
      settings: xl_area=[0, 0, 0, 0, 0, 0, 0]
  Mux : xbsIndex_r3/Mux  inputs=5  precision=Full  arith_type="Signed  (2's comp)"  n_bits=8  bin_pt=2  quantization=Truncate  overflow=Wrap  latency=1  explicit_period=off  period=1  en=off  dbl_ovrd=off  show_param=off  mux_type=off  use_rpm=off  gen_core=off
      settings: xl_area=[0, 0, 0, 0, 0, 0, 0]
  Slice1 : xbsIndex_r3/Slice  mode=Upper Bit Location + Width  nbits=3  bit1=0  base1=MSB of Input  bit0=0  base0=LSB of Input  boolean_output=off  explicit_period=off  period=1  dbl_ovrd=off
  Slice2 : xbsIndex_r3/Slice  mode=Lower Bit Location + Width  nbits=10  bit1=0  base1=MSB of Input  bit0=0  base0=LSB of Input  boolean_output=off  explicit_period=off  period=1  dbl_ovrd=off
  bram0 : xbsIndex_r3/Single Port RAM  depth=1024  initVector=sin(pi*(0:15)/16)  write_mode=Read Before Write  latency=2  init_zero=on  explicit_period=off  period=1  rst=off  init_reg=0  en=off  dbl_ovrd=off  show_param=off  distributed_mem=off  use_rpm=off  gen_core=off
      settings: xl_area=[0, 0, 0, 0, 0, 0, 0]
  delay_d0 : xbsIndex_r3/Delay  latency=4  reg_retiming=off  explicit_period=off  period=1  en=off  accept_only_valid=off  init_zero=on  dbl_ovrd=off  show_param=off
      settings: xl_area=[0, 0, 0, 0, 0, 0, 0]
  delay_din0 : xbsIndex_r3/Delay  latency=5  reg_retiming=off  explicit_period=off  period=1  en=off  accept_only_valid=off  init_zero=on  dbl_ovrd=off  show_param=off
      settings: xl_area=[0, 0, 0, 0, 0, 0, 0]
  delay_map1 : xbsIndex_r3/Delay  latency=3*map_latency  reg_retiming=off  explicit_period=off  period=1  en=off  accept_only_valid=off  init_zero=on  dbl_ovrd=off  show_param=off
      settings: xl_area=[0, 0, 0, 0, 0, 0, 0]
  delay_map2 : xbsIndex_r3/Delay  latency=2*map_latency  reg_retiming=off  explicit_period=off  period=1  en=off  accept_only_valid=off  init_zero=on  dbl_ovrd=off  show_param=off
      settings: xl_area=[0, 0, 0, 0, 0, 0, 0]
  delay_map3 : xbsIndex_r3/Delay  latency=1*map_latency  reg_retiming=off  explicit_period=off  period=1  en=off  accept_only_valid=off  init_zero=on  dbl_ovrd=off  show_param=off
      settings: xl_area=[0, 0, 0, 0, 0, 0, 0]
  delay_map4 : xbsIndex_r3/Delay  latency=0*map_latency  reg_retiming=off  explicit_period=off  period=1  en=off  accept_only_valid=off  init_zero=on  dbl_ovrd=off  show_param=off
      settings: xl_area=[0, 0, 0, 0, 0, 0, 0]
  delay_sel : xbsIndex_r3/Delay  latency=4  reg_retiming=off  explicit_period=off  period=1  en=off  accept_only_valid=off  init_zero=on  dbl_ovrd=off  show_param=off
      settings: xl_area=[0, 0, 0, 0, 0, 0, 0]
  delay_valid : xbsIndex_r3/Delay  latency=3  reg_retiming=off  explicit_period=off  period=1  en=off  accept_only_valid=off  init_zero=on  dbl_ovrd=off  show_param=off
      settings: xl_area=[0, 0, 0, 0, 0, 0, 0]
  delay_we : xbsIndex_r3/Delay  latency=4  reg_retiming=off  explicit_period=off  period=1  en=off  accept_only_valid=off  init_zero=on  dbl_ovrd=off  show_param=off
      settings: xl_area=[0, 0, 0, 0, 0, 0, 0]
  map{1..4} (4 alike) : xbsIndex_r3/ROM  depth=1024  initVector=[0 16 32 48 64 80 96 112 128 144 160 176 192 208 224 240 256 272 288 304 320 336 352 368 384 400 416 432 448 464 480 496 512 528 544 560 576 592 608 624 640 656 672 688 704 720 736 752 768 784 800 816 832 848 864 880 896 912 928 944 960 976 992 1008 1 17 33 49 65 81 97 113 129 145 161 177 193 209 225 241 257 273 289 305 321 337 353 369 385 401 417 433 449 465 481 497 513 529 545 561 577 593 609 625 641 657 673 689 705 721 737 753 769 785 801 817 833 849 865 881 897 913 929 945 961 977 993 1009 2 18 34 50 66 82 98 114 130 146 162 178 194 210 226 242 258 274 290 306 322 338 354 370 386 402 418 434 450 466 482 498 514 530 546 562 578 594 610 626 642 658 674 690 706 722 738 754 770 786 802 818 834 850 866 882 898 914 930 946 962 978 994 1010 3 19 35 51 67 83 99 115 131 147 163 179 195 211 227 243 259 275 291 307 323 339 355 371 387 403 419 435 451 467 483 499 515 531 547 563 579 595 611 627 643 659 675 691 707 723 739 755 771 787 803 819 835 851 867 883 899 915 931 947 963 979 995 1011 4 20 36 52 68 84 100 116 132 148 164 180 196 212 228 244 260 276 292 308 324 340 356 372 388 404 420 436 452 468 484 500 516 532 548 564 580 596 612 628 644 660 676 692 708 724 740 756 772 788 804 820 836 852 868 884 900 916 932 948 964 980 996 1012 5 21 37 53 69 85 101 117 133 149 165 181 197 213 229 245 261 277 293 309 325 341 357 373 389 405 421 437 453 469 485 501 517 533 549 565 581 597 613 629 645 661 677 693 709 725 741 757 773 789 805 821 837 853 869 885 901 917 933 949 965 981 997 1013 6 22 38 54 70 86 102 118 134 150 166 182 198 214 230 246 262 278 294 310 326 342 358 374 390 406 422 438 454 470 486 502 518 534 550 566 582 598 614 630 646 662 678 694 710 726 742 758 774 790 806 822 838 854 870 886 902 918 934 950 966 982 998 1014 7 23 39 55 71 87 103 119 135 151 167 183 199 215 231 247 263 279 295 311 327 343 359 375 391 407 423 439 455 471 487 503 519 535 551 567 583 599 615 631 647 663 679 695 711 727 743 759 775 791 807 823 839 855 871 887 903 919 935 951 967 983 999 1015 8 24 40 56 72 88 104 120 136 152 168 184 200 216 232 248 264 280 296 312 328 344 360 376 392 408 424 440 456 472 488 504 520 536 552 568 584 600 616 632 648 664 680 696 712 728 744 760 776 792 808 824 840 856 872 888 904 920 936 952 968 984 1000 1016 9 25 41 57 73 89 105 121 137 153 169 185 201 217 233 249 265 281 297 313 329 345 361 377 393 409 425 441 457 473 489 505 521 537 553 569 585 601 617 633 649 665 681 697 713 729 745 761 777 793 809 825 841 857 873 889 905 921 937 953 969 985 1001 1017 10 26 42 58 74 90 106 122 138 154 170 186 202 218 234 250 266 282 298 314 330 346 362 378 394 410 426 442 458 474 490 506 522 538 554 570 586 602 618 634 650 666 682 698 714 730 746 762 778 794 810 826 842 858 874 890 906 922 938 954 970 986 1002 1018 11 27 43 59 75 91 107 123 139 155 171 187 203 219 235 251 267 283 299 315 331 347 363 379 395 411 427 443 459 475 491 507 523 539 555 571 587 603 619 635 651 667 683 699 715 731 747 763 779 795 811 827 843 859 875 891 907 923 939 955 971 987 1003 1019 12 28 44 60 76 92 108 124 140 156 172 188 204 220 236 252 268 284 300 316 332 348 364 380 396 412 428 444 460 476 492 508 524 540 556 572 588 604 620 636 652 668 684 700 716 732 748 764 780 796 812 828 844 860 876 892 908 924 940 956 972 988 1004 1020 13 29 45 61 77 93 109 125 141 157 173 189 205 221 237 253 269 285 301 317 333 349 365 381 397 413 429 445 461 477 493 509 525 541 557 573 589 605 621 637 653 669 685 701 717 733 749 765 781 797 813 829 845 861 877 893 909 925 941 957 973 989 1005 1021 14 30 46 62 78 94 110 126 142 158 174 190 206 222 238 254 270 286 302 318 334 350 366 382 398 414 430 446 462 478 494 510 526 542 558 574 590 606 622 638 654 670 686 702 718 734 750 766 782 798 814 830 846 862 878 894 910 926 942 958 974 990 1006 1022 15 31 47 63 79 95 111 127 143 159 175 191 207 223 239 255 271 287 303 319 335 351 367 383 399 415 431 447 463 479 495 511 527 543 559 575 591 607 623 639 655 671 687 703 719 735 751 767 783 799 815 831 847 863 879 895 911 927 943 959 975 991 1007 1023]  arith_type=Unsigned  n_bits=10  bin_pt=0  latency=1  init_zero=on  explicit_period=off  period=1  rst=off  init_reg=0  en=off  dbl_ovrd=off  show_param=off  distributed_mem=on  use_rpm=off  gen_core=off
      settings: xl_area=[0, 0, 0, 0, 0, 0, 0]
  post_sync_delay : xbsIndex_r3/Delay  latency=3  reg_retiming=off  explicit_period=off  period=1  en=off  accept_only_valid=off  init_zero=on  dbl_ovrd=off  show_param=off
      settings: xl_area=[0, 0, 0, 0, 0, 0, 0]
  pre_sync_delay : xbsIndex_r3/Delay  latency=4  reg_retiming=off  explicit_period=off  period=1  en=off  accept_only_valid=off  init_zero=on  dbl_ovrd=off  show_param=off
      settings: xl_area=[0, 0, 0, 0, 0, 0, 0]
  sync_delay_en : casper_library/Delays/sync_delay_en  DelayLen=1024
      link override Constant: equ=P=C
      link override Constant1: equ=P=C
      link override Constant2: equ=P=C
      link override Constant3: equ=P=C
  sync_out : Outport
  valid : Outport  Port=2
  dout0 : Outport  Port=3
  wires:
  sync/1 -> Counter/1, pre_sync_delay/1
  en/1 -> Counter/2, sync_delay_en/2, delay_we/1
  Counter/1 -> Slice1/1, Slice2/1
  Slice1/1 -> delay_sel/1
  delay_sel/1 -> Mux/1
  Slice2/1 -> delay_d0/1, map1/1
  delay_d0/1 -> Mux/2
  pre_sync_delay/1 -> sync_delay_en/1
  sync_delay_en/1 -> post_sync_delay/1
  post_sync_delay/1 -> sync_out/1
  delay_we/1 -> delay_valid/1, bram0/3
  delay_valid/1 -> valid/1
  Mux/1 -> bram0/1
  din0/1 -> delay_din0/1
  delay_din0/1 -> bram0/2
  bram0/1 -> dout0/1
  map1/1 -> delay_map1/1, map2/1
  delay_map1/1 -> Mux/3
  map2/1 -> delay_map2/1, map3/1
  delay_map2/1 -> Mux/4
  map3/1 -> delay_map3/1, map4/1
  delay_map3/1 -> Mux/5
  map4/1 -> delay_map4/1
  delay_map4/1 -> Mux/6
